simulink model "hopper4"  (R2015b)
settings: Solver=ode23s  StartTime=0.0  StopTime=15  MinStep=1e-8  RelTol=1e-3
undefined symbols (not defined in the file): sigbuilder_block, X, Y, Z
libraries: sm_lib x30, nesl_utility x24, Contact_Forces_Lib x1, Parts_Lib x1
(part 2 of 2)

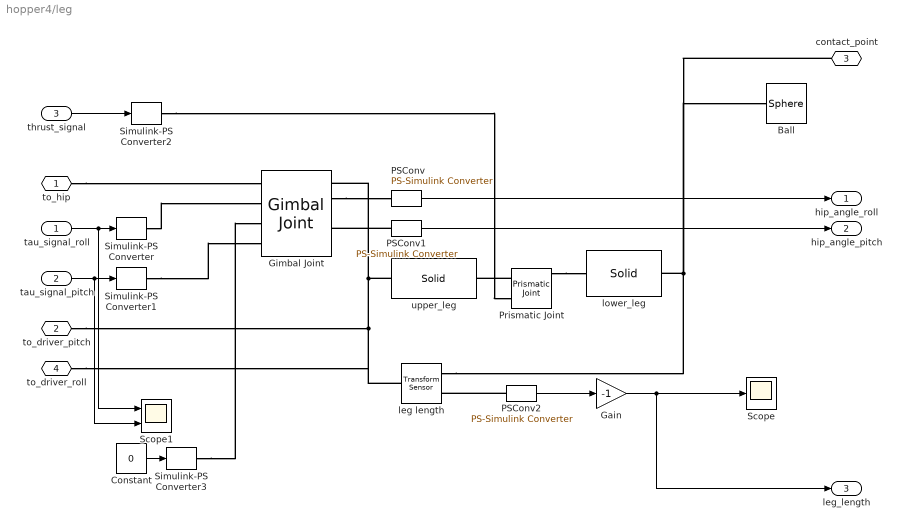
== system hopper4/leg ==
  tau_signal_roll : Inport
  tau_signal_pitch : Inport  Port=2
  thrust_signal : Inport  Port=3
  Ball : Parts_Lib/Sphere  Tag=CustomStyle  sph_radius=0.05  sph_density=1000  sph_color=red  sph_opacity=1  mark_type=Rings on center planes  arc_width=[40 50]  arc_angle=60  ring_width=5  ring_irad=0.95  mark_color=axes  mark_opacity=1  ring_opacity=0  arc_opacity=0
  Constant : Constant  Value=0
  Gain : Gain  Gain=-1
  Gimbal Joint : sm_lib/Joints/Gimbal Joint  SenseConstraintForce=off  SenseConstraintForceX=off  SenseConstraintForceY=off  SenseConstraintForceZ=off  SenseConstraintTorque=off  SenseConstraintTorqueX=off  SenseConstraintTorqueY=off  SenseConstraintTorqueZ=off  SenseTotalForce=off  SenseTotalForceX=off  SenseTotalForceY=off  SenseTotalForceZ=off  SenseTotalTorque=off  SenseTotalTorqueX=off  SenseTotalTorqueY=off  SenseTotalTorqueZ=off  CompositeWrenchDir=FollowerOnBase  CompositeWrenchFrame=BaseFrame  RxEquilibriumPosition=0  RxEquilibriumPositionUnits=deg  RxSpringStiffness=0  RxSpringStiffnessUnits=N*m/deg  RxDampingCoefficient=0.03  RxDampingCoefficientUnits=N*m/(deg/s)  RxTorqueActuationMode=InputTorque  RxMotionActuationMode=ComputedMotion  RxSensePosition=on  RxSenseVelocity=on  RxSenseAcceleration=off  RxSenseTorqueForce=off  RxPositionTargetSpecify=off  RxPositionTargetPriority=High  RxPositionTargetValue=0  RxPositionTargetValueUnits=deg  RxVelocityTargetSpecify=off  RxVelocityTargetPriority=High  RxVelocityTargetValue=0  RxVelocityTargetValueUnits=deg/s  RyEquilibriumPosition=0  RyEquilibriumPositionUnits=deg  RySpringStiffness=0  RySpringStiffnessUnits=N*m/deg  RyDampingCoefficient=0.03  RyDampingCoefficientUnits=N*m/(deg/s)  RyTorqueActuationMode=ComputedTorque  RyMotionActuationMode=InputMotion  RySensePosition=off  RySenseVelocity=off  RySenseAcceleration=off  RySenseTorqueForce=off  RyPositionTargetSpecify=on  RyPositionTargetPriority=High  RyPositionTargetValue=0  RyPositionTargetValueUnits=deg  RyVelocityTargetSpecify=on  RyVelocityTargetPriority=High  RyVelocityTargetValue=0  RyVelocityTargetValueUnits=deg/s  RzEquilibriumPosition=0  RzEquilibriumPositionUnits=deg  RzSpringStiffness=0  RzSpringStiffnessUnits=N*m/deg  RzDampingCoefficient=0.03  RzDampingCoefficientUnits=N*m/(deg/s)  RzTorqueActuationMode=InputTorque  RzMotionActuationMode=ComputedMotion  RzSensePosition=on  RzSenseVelocity=on  RzSenseAcceleration=off  RzSenseTorqueForce=off  RzPositionTargetSpecify=off  RzPositionTargetPriority=High  RzPositionTargetValue=0  RzPositionTargetValueUnits=deg  RzVelocityTargetSpecify=off  RzVelocityTargetPriority=High  RzVelocityTargetValue=0  RzVelocityTargetValueUnits=deg/s  BlockFunction=simmechanics.library.joints.gimbal_joint
  PSConv : nesl_utility/PS-Simulink Converter  PhysicalDomain=network_engine_domain  SubClassName=ps_output  LeftPortType=input  RightPortType=output  PseudoPeriodic=off  Frequencies=[]  Unit=1  AffineConversion=off
  PSConv1 : nesl_utility/PS-Simulink Converter  PhysicalDomain=network_engine_domain  SubClassName=ps_output  LeftPortType=input  RightPortType=output  PseudoPeriodic=off  Frequencies=[]  Unit=1  AffineConversion=off
  PSConv2 : nesl_utility/PS-Simulink Converter  PhysicalDomain=network_engine_domain  SubClassName=ps_output  LeftPortType=input  RightPortType=output  PseudoPeriodic=off  Frequencies=[]  Unit=1  AffineConversion=off
  Prismatic Joint : sm_lib/Joints/Prismatic Joint  SenseConstraintForce=off  SenseConstraintForceX=off  SenseConstraintForceY=off  SenseConstraintForceZ=off  SenseConstraintTorque=off  SenseConstraintTorqueX=off  SenseConstraintTorqueY=off  SenseConstraintTorqueZ=off  SenseTotalForce=off  SenseTotalForceX=off  SenseTotalForceY=off  SenseTotalForceZ=off  SenseTotalTorque=off  SenseTotalTorqueX=off  SenseTotalTorqueY=off  SenseTotalTorqueZ=off  CompositeWrenchDir=FollowerOnBase  CompositeWrenchFrame=BaseFrame  EquilibriumPosition=0  EquilibriumPositionUnits=m  SpringStiffness=7e3  SpringStiffnessUnits=N/m  DampingCoefficient=40  DampingCoefficientUnits=N/(m/s)  TorqueActuationMode=InputTorque  MotionActuationMode=ComputedMotion  SensePosition=on  SenseVelocity=on  SenseAcceleration=off  SenseTorqueForce=off  PositionTargetSpecify=on  PositionTargetPriority=High  PositionTargetValue=0  PositionTargetValueUnits=m  VelocityTargetSpecify=off  VelocityTargetPriority=High  VelocityTargetValue=0  VelocityTargetValueUnits=m/s  BlockFunction=simmechanics.library.joints.prismatic_joint
  Scope : Scope
  Scope1 : Scope  NumInputPorts=2
  Simulink-PS Converter{,1..3} (4 alike) : nesl_utility/Simulink-PS Converter  PhysicalDomain=network_engine_domain  SubClassName=ps_input  LeftPortType=input  RightPortType=output  PseudoPeriodic=off  Frequencies=[]  NoiseDistribution=none  NoiseParameters=[]  Unit=1  AffineConversion=off  InputFiltering=on  SimscapeFilterOrder=2  InputFilterTimeConstant=0.001  UdotUserProvided=1
  leg length : sm_lib/Frames and Transforms/Transform Sensor  MeasurementFrame=Follower  SenseAngle=off  SenseAxis=off  SenseAngle1=off  SenseAngle2=off  SenseAngle3=off  SenseQ=off  SenseR=off  SenseOmegaX=off  SenseOmegaY=off  SenseOmegaZ=off  SenseOmega1=off  SenseOmega2=off  SenseOmega3=off  SenseQDot=off  SenseRDot=off  SenseAlphaX=off  SenseAlphaY=off  SenseAlphaZ=off  SenseAlpha1=off  SenseAlpha2=off  SenseAlpha3=off  SenseQDDot=off  SenseRDDot=off  SenseX=off  SenseY=off  SenseZ=on  SenseRad=off  SenseAzim=off  SenseDist=off  SenseInc=off  SenseXDot=off  SenseYDot=off  SenseZDot=off  SenseRadDot=off  SenseAzimDot=off  SenseDistDot=off  SenseIncDot=off  SenseXDDot=off  SenseYDDot=off  SenseZDDot=off  SenseRadDDot=off  SenseAzimDDot=off  SenseDistDDot=off  SenseIncDDot=off  BlockFunction=simmechanics.library.frames_transforms.transform_sensor
  lower_leg : sm_lib/Body Elements/Solid  InertiaType=CalculateFromGeometry  Mass=1  MassUnits=kg  CenterOfMass=[0 0 0]  CenterOfMassUnits=m  MomentsOfInertia=[1 1 1]  MomentsOfInertiaUnits=kg*m^2  ProductsOfInertia=[0 0 0]  ProductsOfInertiaUnits=kg*m^2  DensityBased=on  Density=660  DensityUnits=kg/(m^3)  DoExposeReferenceFrame=off  SerializedFrames=<Frames><Frame><Id>Frame1</Id><Value><Name>joint_F</Name><Origin><Source>GeometricFeature</Source><FeatureName>+z surface</FeatureName></Origin><PrimaryAxis><DefinedDirection>+Z</DefinedDirection><Source>ReferenceFrame</Source><SourceDirection>+Z</SourceDirection><FeatureName></FeatureName></PrimaryAxis><SecondaryAxis><DefinedDirection>+X</DefinedDirection><Source>ReferenceFrame</Source><SourceDirection>+X</SourceDirection><FeatureName></FeatureName></SecondaryAxis></Value></Frame><Frame><Id>Frame2</Id><Value><Name>td_F</Name><Origin><Source>GeometricFeature</Source><FeatureName>-z surface</FeatureName></Origin><PrimaryAxis><DefinedDirection>+Z</DefinedDirection><Source>ReferenceFrame</Source><SourceDirection>+Z</SourceDirection><FeatureName></FeatureName></PrimaryAxis><SecondaryAxis><DefinedDirection>+X</DefinedDirection><Source>ReferenceFrame</Source><SourceDirection>+X</SourceDirection><FeatureName></FeatureName></SecondaryAxis></Value></Frame></Frames>  GraphicType=FromGeometry  MarkerShape=Sphere  MarkerSize=10  GraphicVisPropType=SimpleVisualProperties  GraphicDiffuseColor=[0.6 0.2 1.0]  GraphicSpecularColor=[0.5 0.5 0.5 1.0]  GraphicAmbientColor=[0.15 0.15 0.15 1.0]  GraphicEmissiveColor=[0.0 0.0 0.0 1.0]  GraphicShininess=75  GraphicOpacity=1.0  GeometryShape=Brick  RectangleSize=[1 1]  RectangleSizeUnits=m  BrickDimensions=[0.04 0.04 0.3]  BrickDimensionUnits=m  CylinderRadius=1  CylinderRadiusUnits=m  CylinderLength=1  CylinderLengthUnits=m  SphereRadius=1  SphereRadiusUnits=m  EllipsoidRadii=[1 1 1]  EllipsoidRadiiUnits=m  ExtrusionCrossSection=[1 1; -1 1; -1 -1; 1 -1]  ExtrusionCrossSectionUnits=m  ExtrusionLength=1  ExtrusionLengthUnits=m  PolygonNumSides=3  PolygonOuterRadius=1  PolygonOuterRadiusUnits=m  ExtGeomFileType=STL  ExtGeomFileUnits=m  RevolutionCrossSection=[1 1; 1 -1; 2 -1; 2 1]  RevolutionCrossSectionUnits=m  RevolutionExtent=Full  RevolutionAngle=180  RevolutionAngleUnits=deg  BlockFunction=simmechanics.library.body_elements.solid
  upper_leg : sm_lib/Body Elements/Solid  InertiaType=CalculateFromGeometry  Mass=1  MassUnits=kg  CenterOfMass=[0 0 0]  CenterOfMassUnits=m  MomentsOfInertia=[1 1 1]  MomentsOfInertiaUnits=kg*m^2  ProductsOfInertia=[0 0 0]  ProductsOfInertiaUnits=kg*m^2  DensityBased=on  Density=660  DensityUnits=kg/(m^3)  DoExposeReferenceFrame=off  SerializedFrames=<Frames><Frame><Id>Frame1</Id><Value><Name>hip_F</Name><Origin><Source>GeometricFeature</Source><FeatureName>+z surface</FeatureName></Origin><PrimaryAxis><DefinedDirection>+Z</DefinedDirection><Source>ReferenceFrame</Source><SourceDirection>-Y</SourceDirection><FeatureName></FeatureName></PrimaryAxis><SecondaryAxis><DefinedDirection>+X</DefinedDirection><Source>ReferenceFrame</Source><SourceDirection>+X</SourceDirection><FeatureName></FeatureName></SecondaryAxis></Value></Frame><Frame><Id>Frame2</Id><Value><Name>joint_F</Name><Origin><Source>GeometricFeature</Source><FeatureName>-z surface</FeatureName></Origin><PrimaryAxis><DefinedDirection>+Z</DefinedDirection><Source>ReferenceFrame</Source><SourceDirection>+Z</SourceDirection><FeatureName></FeatureName></PrimaryAxis><SecondaryAxis><DefinedDirection>+X</DefinedDirection><Source>ReferenceFrame</Source><SourceDirection>+X</SourceDirection><FeatureName></FeatureName></SecondaryAxis></Value></Frame></Frames>  GraphicType=FromGeometry  MarkerShape=Sphere  MarkerSize=10  GraphicVisPropType=SimpleVisualProperties  GraphicDiffuseColor=[0.8 0.0 0.8]  GraphicSpecularColor=[0.5 0.5 0.5 1.0]  GraphicAmbientColor=[0.15 0.15 0.15 1.0]  GraphicEmissiveColor=[0.0 0.0 0.0 1.0]  GraphicShininess=75  GraphicOpacity=1.0  GeometryShape=Brick  RectangleSize=[1 1]  RectangleSizeUnits=m  BrickDimensions=[0.04 0.04 0.3]  BrickDimensionUnits=m  CylinderRadius=1  CylinderRadiusUnits=m  CylinderLength=1  CylinderLengthUnits=m  SphereRadius=1  SphereRadiusUnits=m  EllipsoidRadii=[1 1 1]  EllipsoidRadiiUnits=m  ExtrusionCrossSection=[1 1; -1 1; -1 -1; 1 -1]  ExtrusionCrossSectionUnits=m  ExtrusionLength=1  ExtrusionLengthUnits=m  PolygonNumSides=3  PolygonOuterRadius=1  PolygonOuterRadiusUnits=m  ExtGeomFileType=STL  ExtGeomFileUnits=m  RevolutionCrossSection=[1 1; 1 -1; 2 -1; 2 1]  RevolutionCrossSectionUnits=m  RevolutionExtent=Full  RevolutionAngle=180  RevolutionAngleUnits=deg  BlockFunction=simmechanics.library.body_elements.solid
  to_hip : PMIOPort  Port=1  Side=Left
  to_driver_pitch : PMIOPort  Port=2  Side=Left
  contact_point : PMIOPort  Port=3  Side=Right
  to_driver_roll : PMIOPort  Port=4  Side=Left
  hip_angle_roll : Outport
  hip_angle_pitch : Outport  Port=2
  leg_length : Outport  Port=3
  wires:
  Gain/1 -> leg_length/1, Scope/1
  PSConv2/1 -> Gain/1
  PSConv/1 -> hip_angle_roll/1
  tau_signal_roll/1 -> Scope1/1, Simulink-PS Converter/1
  tau_signal_pitch/1 -> Scope1/2, Simulink-PS Converter1/1
  PSConv1/1 -> hip_angle_pitch/1
  thrust_signal/1 -> Simulink-PS Converter2/1
  Constant/1 -> Simulink-PS Converter3/1
  connections:
  Gimbal Joint/RConn2 -- PSConv/LConn1
  Prismatic Joint/RConn1 -- lower_leg/LConn1
  contact_point/RConn1 -- Ball/LConn1 -- leg length/RConn1 -- lower_leg/RConn1
  upper_leg/LConn1 -- to_driver_roll/RConn1 -- leg length/LConn1 -- to_driver_pitch/RConn1 -- Gimbal Joint/RConn1
  Prismatic Joint/LConn1 -- upper_leg/RConn1
  to_hip/RConn1 -- Gimbal Joint/LConn1
  PSConv2/LConn1 -- leg length/RConn2
  Simulink-PS Converter/RConn1 -- Gimbal Joint/LConn2
  Simulink-PS Converter1/RConn1 -- Gimbal Joint/LConn4
  PSConv1/LConn1 -- Gimbal Joint/RConn4
  Simulink-PS Converter2/RConn1 -- Prismatic Joint/LConn2
  Simulink-PS Converter3/RConn1 -- Gimbal Joint/LConn3

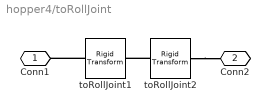
== system hopper4/toRollJoint ==
  toRollJoint1 : sm_lib/Frames and Transforms/Rigid Transform  TranslationMethod=Cartesian  TranslationLengthUnit=m  TranslationStandardAxis=+Z  TranslationStandardOffset=0  TranslationCartesianOffset=[0 0.1 -0.1]  TranslationROffset=0  TranslationROffsetUnits=m  TranslationZOffset=0  TranslationZOffsetUnits=m  TranslationThetaOffset=0  TranslationThetaOffsetUnits=deg  RotationMethod=None  RotationAngleUnits=deg  RotationStandardAxis=+Z  RotationAngle=0.0  RotationArbitraryAxis=[0 0 1]  FollAlignAxisA=+X  BaseAlignAxisA=+Y  FollAlignAxisB=+Y  BaseAlignAxisB=+Z  RotationSequenceAxes=FollowerAxes  RotationSequence=XYX  RotationSequenceAngles=[0 0 0]  RotationSequenceAnglesUnits=deg  RotationMatrix=[1 0 0; 0 1 0; 0 0 1]  BlockFunction=simmechanics.library.frames_transforms.rigid_transform
  toRollJoint2 : sm_lib/Frames and Transforms/Rigid Transform  TranslationMethod=None  TranslationLengthUnit=m  TranslationStandardAxis=+Z  TranslationStandardOffset=0  TranslationCartesianOffset=[0 0.1 -0.1]  TranslationROffset=0  TranslationROffsetUnits=m  TranslationZOffset=0  TranslationZOffsetUnits=m  TranslationThetaOffset=0  TranslationThetaOffsetUnits=deg  RotationMethod=AlignedAxes  RotationAngleUnits=deg  RotationStandardAxis=+Z  RotationAngle=0.0  RotationArbitraryAxis=[0 0 1]  FollAlignAxisA=+Y  BaseAlignAxisA=+Y  FollAlignAxisB=+X  BaseAlignAxisB=+Z  RotationSequenceAxes=FollowerAxes  RotationSequence=XYX  RotationSequenceAngles=[0 0 0]  RotationSequenceAnglesUnits=deg  RotationMatrix=[1 0 0; 0 1 0; 0 0 1]  BlockFunction=simmechanics.library.frames_transforms.rigid_transform
  Conn1 : PMIOPort  Port=1  Side=Left
  Conn2 : PMIOPort  Port=2  Side=Right
  connections:
  toRollJoint2/LConn1 -- toRollJoint1/RConn1
  toRollJoint1/LConn1 -- Conn1/RConn1
  toRollJoint2/RConn1 -- Conn2/RConn1

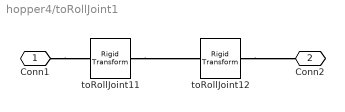
== system hopper4/toRollJoint1 ==
  toRollJoint11 : sm_lib/Frames and Transforms/Rigid Transform  TranslationMethod=None  TranslationLengthUnit=m  TranslationStandardAxis=+Z  TranslationStandardOffset=0  TranslationCartesianOffset=[0 0.1 0]  TranslationROffset=0  TranslationROffsetUnits=m  TranslationZOffset=0  TranslationZOffsetUnits=m  TranslationThetaOffset=0  TranslationThetaOffsetUnits=deg  RotationMethod=AlignedAxes  RotationAngleUnits=deg  RotationStandardAxis=+Z  RotationAngle=0.0  RotationArbitraryAxis=[0 0 1]  FollAlignAxisA=+Y  BaseAlignAxisA=+Y  FollAlignAxisB=+X  BaseAlignAxisB=-Z  RotationSequenceAxes=FollowerAxes  RotationSequence=XYX  RotationSequenceAngles=[0 0 0]  RotationSequenceAnglesUnits=deg  RotationMatrix=[1 0 0; 0 1 0; 0 0 1]  BlockFunction=simmechanics.library.frames_transforms.rigid_transform
  toRollJoint12 : sm_lib/Frames and Transforms/Rigid Transform  TranslationMethod=Cartesian  TranslationLengthUnit=m  TranslationStandardAxis=+Z  TranslationStandardOffset=0  TranslationCartesianOffset=[0 0.1 0]  TranslationROffset=0  TranslationROffsetUnits=m  TranslationZOffset=0  TranslationZOffsetUnits=m  TranslationThetaOffset=0  TranslationThetaOffsetUnits=deg  RotationMethod=None  RotationAngleUnits=deg  RotationStandardAxis=+Z  RotationAngle=0.0  RotationArbitraryAxis=[0 0 1]  FollAlignAxisA=+X  BaseAlignAxisA=+Y  FollAlignAxisB=+Y  BaseAlignAxisB=+Z  RotationSequenceAxes=FollowerAxes  RotationSequence=XYX  RotationSequenceAngles=[0 0 0]  RotationSequenceAnglesUnits=deg  RotationMatrix=[1 0 0; 0 1 0; 0 0 1]  BlockFunction=simmechanics.library.frames_transforms.rigid_transform
  Conn1 : PMIOPort  Port=1  Side=Left
  Conn2 : PMIOPort  Port=2  Side=Right
  connections:
  Conn1/RConn1 -- toRollJoint11/LConn1
  toRollJoint12/RConn1 -- Conn2/RConn1
  toRollJoint11/RConn1 -- toRollJoint12/LConn1

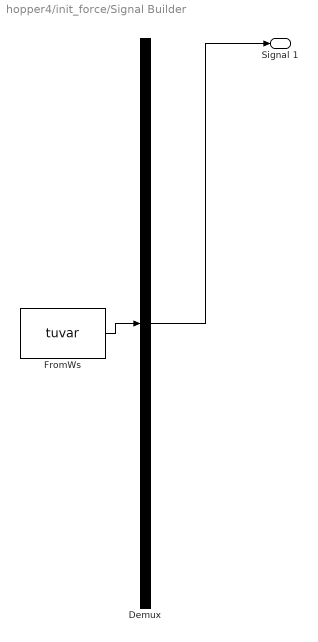
== system hopper4/init_force/Signal Builder ==
  Demux : Demux  Tag=STV Demux  Outputs=1
  FromWs : FromWorkspace  Tag=STV FromWs  VariableName=tuvar  SampleTime=0
      SigBuilderData=|
      | common.afterFinalStr = 'Extrapolate'
      | common.sampleTime = 0
      | dataSet.timeRange = [0 10]
      | dataSet.name = 'Group 1'
      | sbobj.Groups.Name = 'Group 1'
      | sbobj.Groups.Signals.Name = 'Signal 1'
      | sbobj.Groups.Signals.XData = [0 1 1 1.34 1.34 10]
      | sbobj.Groups.Signals.YData = [0 0 7.3 7.3 0 0]
  Signal 1 : Outport  Tag=STV Outport
  wires:
  Demux/1 -> Signal 1/1
  FromWs/1 -> Demux/1

== matlab function hopper4/MATLAB Function ==
  data: state input; thrust output
function thrust = thrust_input(state)
%#codegen

if state == 4
    thrust = -660;
else
    thrust = 0;
end

== matlab function hopper4/Contact/MATLAB Function ==
  data: contact_f input; state output; z input; zdot input
function state = state_check(contact_f, z, zdot)
%#codegen

state = 0;
TOUCH_DOWN_HEIGHT = 0.065;% this is an empirical value

if z > TOUCH_DOWN_HEIGHT && zdot > 5e-2 
    % leaving to flight
    state = 1;
elseif z > TOUCH_DOWN_HEIGHT && zdot < -5e-2
    % ready to touchdown
    state = 2;
elseif z > TOUCH_DOWN_HEIGHT && abs(zdot) <= 5e-2
    % slow flight
    state = 3;
 
elseif z <= TOUCH_DOWN_HEIGHT 
    % touch down
    state = 4;
    
end

    
end

== matlab function hopper4/leg_movement_generation ==
  data: drive_length_pitch output; state input; q_fb input; w_pitch input; w_roll input; vx input; vy input; leg_length input; hip_torque_pitch output; drive_length_roll output; hip_torque_roll output; body_angle_y output; body_angle_x output; v_des_x input; v_des_y input
function [drive_length_pitch, hip_torque_pitch,...
    drive_length_roll, hip_torque_roll, ...
    body_angle_y,body_angle_x]= drive_angle(state, ...
    q_fb, w_pitch, w_roll,vx,vy, leg_length, v_des_x, v_des_y)

coder.extrinsic('quatrotate');
coder.extrinsic('quatconj');
coder.extrinsic('quat2eul');
L = 0.1;

Tst = 178.84*0.001; %ms


k_foot = 0.06;
k_p2 =  8;
k_v =  8;

qw = q_fb(1);
qx = q_fb(2);
qy = q_fb(3);
qz = q_fb(4);
%eulZYX = quat2eul(q_fb');
aSinInput = -2*(qx.*qz-qw.*qy);
        aSinInput(aSinInput > 1) = 1;
eulZYX =[ atan2( 2*(qx.*qy+qw.*qz), qw.^2 + qx.^2 - qy.^2 - qz.^2 ), ...
            asin( aSinInput ), ...
            atan2( 2*(qy.*qz+qw.*qx), qw.^2 - qx.^2 - qy.^2 + qz.^2 )];
% eulZYX = zeros(1,3);
% eulZYX = quat2eul(q_fb');
body_angle_y = eulZYX(2);
body_angle_x = eulZYX(3);

if body_angle_y > pi
    body_angle_y = body_angle_y - 2*pi;
elseif body_angle_y < -pi
    body_angle_y = body_angle_y + 2*pi;
end
if body_angle_x > pi
    body_angle_x = body_angle_x - 2*pi;
elseif body_angle_x < -pi
    body_angle_x = body_angle_x + 2*pi;
end

if state ~= 4 
    xf = sqrt(vx*vx + vy*vy)*Tst/2 ; 
    if xf > leg_length
        xf = leg_length;
    elseif xf < -leg_length
        xf = -leg_length;
    end
    % 2016-9-5 need to change frame of xf
    if abs(body_angle_y) > 1e-2 || abs(body_angle_x) > 1e-2
        % 2016-9-14 add direction
        xf = vx *Tst/2 + k_foot*(v_des_x-vx);
        yf = vy *Tst/2 + k_foot*(v_des_y-vy);
        k = sqrt(xf*xf+yf*yf);
        if k > leg_length
            k = leg_length;
        elseif k < -leg_length
            k = -leg_length;
        end
        alpha = asin(k/leg_length);
        
        xf_vec = [xf yf -k/tan(alpha)];
        % xf_vec = [xf*vx/sqrt(vx*vx + vy*vy) xf*vy/sqrt(vx*vx + vy*vy) -xf/tan(alpha)];
        xf_vec_f = zeros(1,3);
        % xf_vec_f = quatrotate(quatconj(q_fb'),xf_vec);
        xf_vec_f = quatrotate(q_fb',xf_vec);
        vx_f = xf_vec_f(1);
        vy_f = xf_vec_f(2);
        r = L/leg_length* sqrt(vx_f*vx_f + vy_f*vy_f);
        theta = atan2(vy_f,-vx_f);
    else
        r = L/leg_length* xf;
        theta = atan2(vy,-vx);
    end
    
    % drive pitch and roll from r and theta
    rhs = L / sqrt(r*r+L*L);
    drive_length_pitch = sqrt(rhs*(-2*L*r*cos(theta)-2*L*L)+3*L*L);
    drive_length_roll = sqrt(rhs*(-2*L*r*cos(pi/2-theta)-2*L*L)+3*L*L);
    hip_torque_pitch = 0.0;
    hip_torque_roll = 0.0;
       
elseif state == 4 && leg_length < 0.55 % empirical value
    drive_length_pitch = -999;
    drive_length_roll = -999;

    hip_torque_pitch = k_p2* (0 - body_angle_y) + k_v * w_pitch;
    hip_torque_pitch = - hip_torque_pitch;
    % pitch torque 1, body_angle_y > 0, w_pitch > 0

    hip_torque_roll = k_p2* (body_angle_x - 0) - k_v * w_roll;
    hip_torque_roll = - hip_torque_roll;
    % roll torque 1, body_angle_x < 0, w_roll < 0

else
    drive_length_pitch = -999;
    drive_length_roll = -999;
    hip_torque_pitch = 0.0;
    hip_torque_roll = 0.0;
end
    %saturation
%     if hip_torque1 > 4
%         hip_torque1 = 4;
%     elseif hip_torque1 < -4
%         hip_torque1 = -4;
%     end
%     if hip_torque2 > 4
%         hip_torque2 = 4;
%     elseif hip_torque2 < -4
%         hip_torque2 = -4;
%     end
end

== matlab function hopper4/driver_pitch/MATLAB Function ==
  data: desire_length input; force output; curr_length input; curr_vel input
function force = length_controller(desire_length, curr_length, curr_vel)
%#codegen
kp = 9500;
kd = 115;

force = 0;
if desire_length == -999
    force = 0;
else
    force = kp*(desire_length-curr_length) - kd*curr_vel;
end

== matlab function hopper4/driver_roll/MATLAB Function ==
  data: desire_length input; force output; curr_length input; curr_vel input
function force = length_controller(desire_length, curr_length, curr_vel)
%#codegen
kp = 9500;
kd = 115;

force = 0;
if desire_length == -999
    force = 0;
else
    force = kp*(desire_length-curr_length) - kd*curr_vel;
end

== matlab function hopper4/velocity_generation ==
  data: pos_x input; v_des_x output; pos_y input; v_des_y output
function [v_des_x, v_des_y] = fcn(pos_x, pos_y)
%#codegen
persistent v_x v_y
if isempty(v_x) 
    v_x = 0.05;
end
if isempty(v_y) 
    v_y = 0;
end

if pos_x > 3
    v_x = 0.05;
elseif pos_x < -3
    v_x = -0.05;
end

v_des_x = v_x;
v_des_y = v_y;
